simulink library "Input_Air"  (Simulink 8.2)
settings: Solver=ode45  StartTime=0.0  StopTime=10.0  RelTol=1e-3
settings Model: Creator=lena.frank  LastModifiedBy=drhf

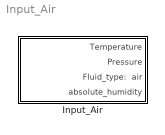
== system Input_Air ==
  Input_Air : Subsystem  mask(Input_Air){T=20, p=1e5, x=0.005}
      mask prompts: T "temperature (scalar or vector) [°C]"; p "pressure [Pa]"; x "absolute humidity of moist air [kg water/kg dry air]"
      mask help:
      | Input block for the material "Air"
      |
      | The relevant inputs for the calculation of the block can be specified as parameter in the mask
      mask Help: web(fullfile(path_carnot('help'),'input_material.html'),'-helpbrowser')

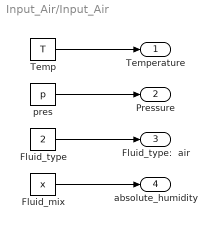
== system Input_Air/Input_Air ==
  Fluid_mix : Constant  Value=x
  Fluid_type : Constant  Value=2
  Temp : Constant  Value=T
  pres : Constant  Value=p
  Temperature : Outport
  Pressure : Outport  Port=2
  Fluid_type:  air : Outport  Port=3
  absolute_humidity : Outport  Port=4
  wires:
  pres/1 -> Pressure/1
  Temp/1 -> Temperature/1
  Fluid_type/1 -> Fluid_type:  air/1
  Fluid_mix/1 -> absolute_humidity/1
